simulink model "untitled"  (R2023b)
settings: Solver=FixedStepAuto  StartTime=0.0  StopTime=tf  FixedStep=T  RelTol=1e-3
values from neighbouring files (symbols this model uses):
  alpha = 0.2    [mainvVers2.m]
  delta = 0.1    [Controllore.m]    (also in Kalman.m; gian.m; main.m; mainvVers2.m)
  x0 = [0 0 0 0]'    [Controllore.m]    (also in Kalman.m = [0 0 0]'; gian.m = [0 0 0]'; main.m = [0 0 0]')
settings Model: Creator=achil  LastModifiedBy=achil
settings OptimizationCC: BlockReduction=off  DefaultParameterBehavior=Inlined  BufferReuse=off

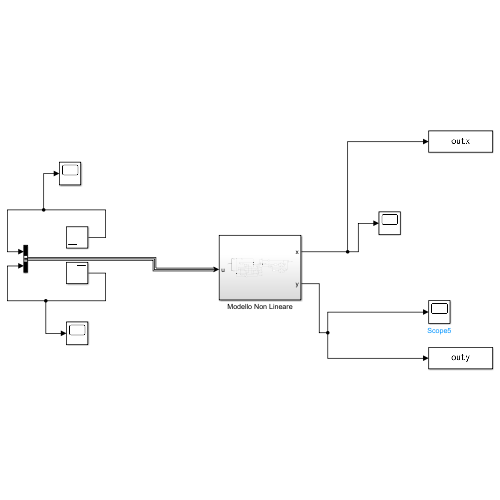
[thumbnail: Simulink's stored preview of the top-level diagram]
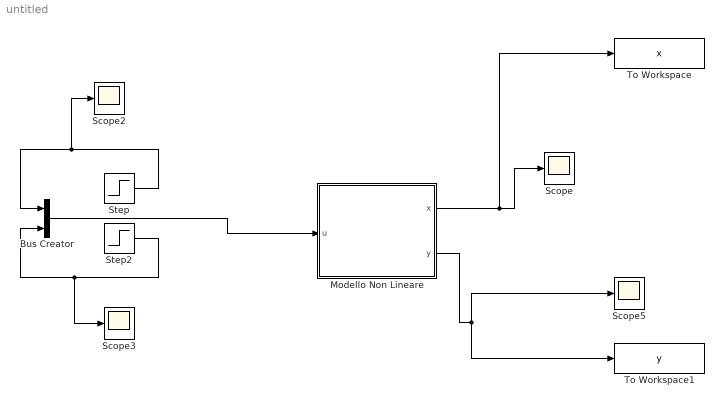
== system untitled ==
  Bus Creator : BusCreator  Inputs=2
  Modello Non Lineare : Subsystem
  Scope{,2..3,5} (4 alike) : Scope
  Step : Step  SampleTime=0
  Step2 : Step  SampleTime=0
  To Workspace : ToWorkspace  VariableName=x  SampleTime=-1
  To Workspace1 : ToWorkspace  VariableName=y  SampleTime=-1
  wires:
  Modello Non Lineare/1(x) -> Scope/1, To Workspace/1
  Step/1 -> Scope2/1, Bus Creator/1
  Step2/1 -> Bus Creator/2, Scope3/1
  Modello Non Lineare/2(y) -> To Workspace1/1, Scope5/1
  Bus Creator/1 -> Modello Non Lineare/1(u)

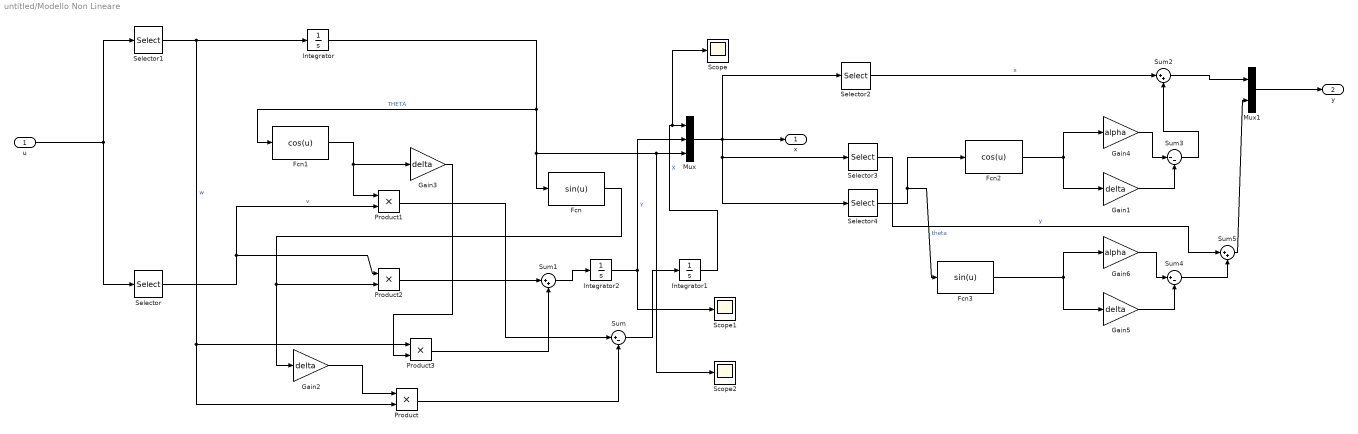
== system untitled/Modello Non Lineare ==
  u : Inport
  Fcn : Fcn  Expr=sin(u)
  Fcn1 : Fcn  Expr=cos(u)
  Fcn2 : Fcn  Expr=cos(u)
  Fcn3 : Fcn  Expr=sin(u)
  Gain{1..3,5} (4 alike) : Gain  Gain=delta
  Gain4 : Gain  Gain=alpha
  Gain6 : Gain  Gain=alpha
  Integrator : Integrator  InitialCondition=x0(3)
  Integrator1 : Integrator  InitialCondition=x0(2)
  Integrator2 : Integrator  InitialCondition=x0(2)
  Mux : Mux  Inputs=3
  Mux1 : Mux  Inputs=2
  Product{,1..3} (4 alike) : Product
  Scope : Scope
  Scope1 : Scope
  Scope2 : Scope
  Selector : Selector  InputPortWidth=2  IndexOptions=Index vector (dialog)  Indices=1  OutputSizes=1
  Selector1 : Selector  InputPortWidth=2  IndexOptions=Index vector (dialog)  Indices=2  OutputSizes=1
  Selector2 : Selector  InputPortWidth=3  IndexOptions=Index vector (dialog)  Indices=1  OutputSizes=1
  Selector3 : Selector  InputPortWidth=3  IndexOptions=Index vector (dialog)  Indices=2  OutputSizes=1
  Selector4 : Selector  InputPortWidth=3  IndexOptions=Index vector (dialog)  Indices=3  OutputSizes=1
  Sum : Sum  Inputs=|+-
  Sum1 : Sum  Inputs=|++
  Sum2 : Sum  Inputs=|++
  Sum3 : Sum  Inputs=|--
  Sum4 : Sum  Inputs=|+-
  Sum5 : Sum  Inputs=|++
  x : Outport
  y : Outport  Port=2
  wires:
  Fcn/1 -> Gain2/1, Product2/2
  Selector1/1 -> Product3/1, Product/2, Integrator/1  "w"
  Integrator/1 -> Fcn/1, Scope2/1, Mux/3, Fcn1/1  "THETA"
  Mux/1 -> Selector4/1, Selector3/1, Selector2/1, x/1
  Integrator1/1 -> Scope/1, Mux/1  "X"
  Selector/1 -> Product2/1, Product1/2  "v"
  Product3/1 -> Sum1/2
  Fcn1/1 -> Product1/1, Gain3/1
  u/1 -> Selector1/1, Selector/1
  Product/1 -> Sum/2
  Sum1/1 -> Integrator2/1
  Integrator2/1 -> Mux/2, Scope1/1  "Y"
  Product1/1 -> Sum/1
  Product2/1 -> Sum1/1
  Gain3/1 -> Product3/2
  Sum/1 -> Integrator1/1
  Gain2/1 -> Product/1
  Selector4/1 -> Fcn3/1, Fcn2/1  "theta"
  Fcn2/1 -> Gain4/1, Gain1/1
  Gain1/1 -> Sum3/2
  Gain4/1 -> Sum3/1
  Selector2/1 -> Sum2/1  "x"
  Sum3/1 -> Sum2/2
  Sum2/1 -> Mux1/1
  Fcn3/1 -> Gain6/1, Gain5/1
  Gain6/1 -> Sum4/1
  Gain5/1 -> Sum4/2
  Selector3/1 -> Sum5/1  "y"
  Sum4/1 -> Sum5/2
  Sum5/1 -> Mux1/2
  Mux1/1 -> y/1
